simulink model "DA42HoloLensForwarder"  (R2021a)
settings: Solver=ode4  StartTime=0.0  StopTime=inf  FixedStep=0.001  RelTol=1e-3
undefined symbols (not defined in the file): Global_Sample_Time
libraries: simulink_extras x5, slrealtimeutilitieslib x2, dspnetwork x1
(part 3 of 5)

== system DA42HoloLensForwarder/FTD_Output_w_Multicast_XPCmod/Hardware_Switches/PanelAndLegroomSwitches/Decode_Flag1 ==
  Coded_Value : Inport
  Bitmask_Value : Constant  Value=hex2dec(Bitmask_Value)
  Bitwise Operator1 : S-Function  FunctionName=sfix_bitop  Parameters=UseBitMask,NumInputPorts,BitMask,BitMaskRealWorld,logicop  SFunctionDeploymentMode=off  EnableBusSupport=off  mask(Bitwise Operator){logicop=AND, UseBitMask=off, NumInputPorts=2, BitMask=bin2dec('11011001'), BitMaskRealWorld=Stored Integer}
      mask prompts: logicop "Operator:"; UseBitMask "Use bit mask ..."; NumInputPorts "Number of input ports:"; BitMask "Bit Mask"; BitMaskRealWorld "Treat mask as:"
      mask help: Perform the specified bitwise operation on the inputs. The output data type should represent zero exactly.
      mask init: same as DA42HoloLensForwarder/FTD_Output_w_Multicast_XPCmod/Hardware_Switches/MiscSwitches/Decode_Flag/Bitwise Operator1
      mask TypeOptions logicop: AND | OR | NAND | NOR | XOR | NOT
      mask Callback logicop: fixptdialog(gcbh)
      mask Callback UseBitMask: fixptdialog(gcbh)
      mask TypeOptions BitMaskRealWorld: Real World Value | Stored Integer
      mask Display: fprintf(['Bitwise\n',logicop,'\n',str])
  Data Type Conversion1 : DataTypeConversion  OutDataTypeStr=uint32
  Data Type Conversion2 : DataTypeConversion  OutDataTypeStr=double
  Data Type Conversion9 : DataTypeConversion  OutDataTypeStr=uint32
  Divide : Product  Inputs=*/
  Flag : Outport
  wires:
  Data Type Conversion2/1 -> Flag/1
  Divide/1 -> Data Type Conversion2/1
  Data Type Conversion1/1 -> Divide/2, Bitwise Operator1/2
  Data Type Conversion9/1 -> Bitwise Operator1/1
  Bitwise Operator1/1 -> Divide/1
  Bitmask_Value/1 -> Data Type Conversion1/1
  Coded_Value/1 -> Data Type Conversion9/1

== system DA42HoloLensForwarder/FTD_Output_w_Multicast_XPCmod/Hardware_Switches/PanelAndLegroomSwitches/Decode_Flag10 ==
  Coded_Value : Inport
  Bitmask_Value : Constant  Value=hex2dec(Bitmask_Value)
  Bitwise Operator1 : S-Function  FunctionName=sfix_bitop  Parameters=UseBitMask,NumInputPorts,BitMask,BitMaskRealWorld,logicop  SFunctionDeploymentMode=off  EnableBusSupport=off  mask(Bitwise Operator){logicop=AND, UseBitMask=off, NumInputPorts=2, BitMask=bin2dec('11011001'), BitMaskRealWorld=Stored Integer}
      mask prompts: logicop "Operator:"; UseBitMask "Use bit mask ..."; NumInputPorts "Number of input ports:"; BitMask "Bit Mask"; BitMaskRealWorld "Treat mask as:"
      mask help: Perform the specified bitwise operation on the inputs. The output data type should represent zero exactly.
      mask init: same as DA42HoloLensForwarder/FTD_Output_w_Multicast_XPCmod/Hardware_Switches/MiscSwitches/Decode_Flag/Bitwise Operator1
      mask TypeOptions logicop: AND | OR | NAND | NOR | XOR | NOT
      mask Callback logicop: fixptdialog(gcbh)
      mask Callback UseBitMask: fixptdialog(gcbh)
      mask TypeOptions BitMaskRealWorld: Real World Value | Stored Integer
      mask Display: fprintf(['Bitwise\n',logicop,'\n',str])
  Data Type Conversion1 : DataTypeConversion  OutDataTypeStr=uint32
  Data Type Conversion2 : DataTypeConversion  OutDataTypeStr=double
  Data Type Conversion9 : DataTypeConversion  OutDataTypeStr=uint32
  Divide : Product  Inputs=*/
  Flag : Outport
  wires:
  Data Type Conversion2/1 -> Flag/1
  Divide/1 -> Data Type Conversion2/1
  Data Type Conversion1/1 -> Divide/2, Bitwise Operator1/2
  Data Type Conversion9/1 -> Bitwise Operator1/1
  Bitwise Operator1/1 -> Divide/1
  Bitmask_Value/1 -> Data Type Conversion1/1
  Coded_Value/1 -> Data Type Conversion9/1

== system DA42HoloLensForwarder/FTD_Output_w_Multicast_XPCmod/Hardware_Switches/PanelAndLegroomSwitches/Decode_Flag11 ==
  Coded_Value : Inport
  Bitmask_Value : Constant  Value=hex2dec(Bitmask_Value)
  Bitwise Operator1 : S-Function  FunctionName=sfix_bitop  Parameters=UseBitMask,NumInputPorts,BitMask,BitMaskRealWorld,logicop  SFunctionDeploymentMode=off  EnableBusSupport=off  mask(Bitwise Operator){logicop=AND, UseBitMask=off, NumInputPorts=2, BitMask=bin2dec('11011001'), BitMaskRealWorld=Stored Integer}
      mask prompts: logicop "Operator:"; UseBitMask "Use bit mask ..."; NumInputPorts "Number of input ports:"; BitMask "Bit Mask"; BitMaskRealWorld "Treat mask as:"
      mask help: Perform the specified bitwise operation on the inputs. The output data type should represent zero exactly.
      mask init: same as DA42HoloLensForwarder/FTD_Output_w_Multicast_XPCmod/Hardware_Switches/MiscSwitches/Decode_Flag/Bitwise Operator1
      mask TypeOptions logicop: AND | OR | NAND | NOR | XOR | NOT
      mask Callback logicop: fixptdialog(gcbh)
      mask Callback UseBitMask: fixptdialog(gcbh)
      mask TypeOptions BitMaskRealWorld: Real World Value | Stored Integer
      mask Display: fprintf(['Bitwise\n',logicop,'\n',str])
  Data Type Conversion1 : DataTypeConversion  OutDataTypeStr=uint32
  Data Type Conversion2 : DataTypeConversion  OutDataTypeStr=double
  Data Type Conversion9 : DataTypeConversion  OutDataTypeStr=uint32
  Divide : Product  Inputs=*/
  Flag : Outport
  wires:
  Coded_Value/1 -> Data Type Conversion9/1
  Bitmask_Value/1 -> Data Type Conversion1/1
  Bitwise Operator1/1 -> Divide/1
  Data Type Conversion9/1 -> Bitwise Operator1/1
  Data Type Conversion1/1 -> Bitwise Operator1/2, Divide/2
  Divide/1 -> Data Type Conversion2/1
  Data Type Conversion2/1 -> Flag/1

== system DA42HoloLensForwarder/FTD_Output_w_Multicast_XPCmod/Hardware_Switches/PanelAndLegroomSwitches/Decode_Flag12 ==
  Coded_Value : Inport
  Bitmask_Value : Constant  Value=hex2dec(Bitmask_Value)
  Bitwise Operator1 : S-Function  FunctionName=sfix_bitop  Parameters=UseBitMask,NumInputPorts,BitMask,BitMaskRealWorld,logicop  SFunctionDeploymentMode=off  EnableBusSupport=off  mask(Bitwise Operator){logicop=AND, UseBitMask=off, NumInputPorts=2, BitMask=bin2dec('11011001'), BitMaskRealWorld=Stored Integer}
      mask prompts: logicop "Operator:"; UseBitMask "Use bit mask ..."; NumInputPorts "Number of input ports:"; BitMask "Bit Mask"; BitMaskRealWorld "Treat mask as:"
      mask help: Perform the specified bitwise operation on the inputs. The output data type should represent zero exactly.
      mask init: same as DA42HoloLensForwarder/FTD_Output_w_Multicast_XPCmod/Hardware_Switches/MiscSwitches/Decode_Flag/Bitwise Operator1
      mask TypeOptions logicop: AND | OR | NAND | NOR | XOR | NOT
      mask Callback logicop: fixptdialog(gcbh)
      mask Callback UseBitMask: fixptdialog(gcbh)
      mask TypeOptions BitMaskRealWorld: Real World Value | Stored Integer
      mask Display: fprintf(['Bitwise\n',logicop,'\n',str])
  Data Type Conversion1 : DataTypeConversion  OutDataTypeStr=uint32
  Data Type Conversion2 : DataTypeConversion  OutDataTypeStr=double
  Data Type Conversion9 : DataTypeConversion  OutDataTypeStr=uint32
  Divide : Product  Inputs=*/
  Flag : Outport
  wires:
  Data Type Conversion2/1 -> Flag/1
  Divide/1 -> Data Type Conversion2/1
  Data Type Conversion1/1 -> Divide/2, Bitwise Operator1/2
  Data Type Conversion9/1 -> Bitwise Operator1/1
  Bitwise Operator1/1 -> Divide/1
  Bitmask_Value/1 -> Data Type Conversion1/1
  Coded_Value/1 -> Data Type Conversion9/1

== system DA42HoloLensForwarder/FTD_Output_w_Multicast_XPCmod/Hardware_Switches/PanelAndLegroomSwitches/Decode_Flag13 ==
  Coded_Value : Inport
  Bitmask_Value : Constant  Value=hex2dec(Bitmask_Value)
  Bitwise Operator1 : S-Function  FunctionName=sfix_bitop  Parameters=UseBitMask,NumInputPorts,BitMask,BitMaskRealWorld,logicop  SFunctionDeploymentMode=off  EnableBusSupport=off  mask(Bitwise Operator){logicop=AND, UseBitMask=off, NumInputPorts=2, BitMask=bin2dec('11011001'), BitMaskRealWorld=Stored Integer}
      mask prompts: logicop "Operator:"; UseBitMask "Use bit mask ..."; NumInputPorts "Number of input ports:"; BitMask "Bit Mask"; BitMaskRealWorld "Treat mask as:"
      mask help: Perform the specified bitwise operation on the inputs. The output data type should represent zero exactly.
      mask init: same as DA42HoloLensForwarder/FTD_Output_w_Multicast_XPCmod/Hardware_Switches/MiscSwitches/Decode_Flag/Bitwise Operator1
      mask TypeOptions logicop: AND | OR | NAND | NOR | XOR | NOT
      mask Callback logicop: fixptdialog(gcbh)
      mask Callback UseBitMask: fixptdialog(gcbh)
      mask TypeOptions BitMaskRealWorld: Real World Value | Stored Integer
      mask Display: fprintf(['Bitwise\n',logicop,'\n',str])
  Data Type Conversion1 : DataTypeConversion  OutDataTypeStr=uint32
  Data Type Conversion2 : DataTypeConversion  OutDataTypeStr=double
  Data Type Conversion9 : DataTypeConversion  OutDataTypeStr=uint32
  Divide : Product  Inputs=*/
  Flag : Outport
  wires:
  Coded_Value/1 -> Data Type Conversion9/1
  Bitmask_Value/1 -> Data Type Conversion1/1
  Bitwise Operator1/1 -> Divide/1
  Data Type Conversion9/1 -> Bitwise Operator1/1
  Data Type Conversion1/1 -> Bitwise Operator1/2, Divide/2
  Divide/1 -> Data Type Conversion2/1
  Data Type Conversion2/1 -> Flag/1

== system DA42HoloLensForwarder/FTD_Output_w_Multicast_XPCmod/Hardware_Switches/PanelAndLegroomSwitches/Decode_Flag14 ==
  Coded_Value : Inport
  Bitmask_Value : Constant  Value=hex2dec(Bitmask_Value)
  Bitwise Operator1 : S-Function  FunctionName=sfix_bitop  Parameters=UseBitMask,NumInputPorts,BitMask,BitMaskRealWorld,logicop  SFunctionDeploymentMode=off  EnableBusSupport=off  mask(Bitwise Operator){logicop=AND, UseBitMask=off, NumInputPorts=2, BitMask=bin2dec('11011001'), BitMaskRealWorld=Stored Integer}
      mask prompts: logicop "Operator:"; UseBitMask "Use bit mask ..."; NumInputPorts "Number of input ports:"; BitMask "Bit Mask"; BitMaskRealWorld "Treat mask as:"
      mask help: Perform the specified bitwise operation on the inputs. The output data type should represent zero exactly.
      mask init: same as DA42HoloLensForwarder/FTD_Output_w_Multicast_XPCmod/Hardware_Switches/MiscSwitches/Decode_Flag/Bitwise Operator1
      mask TypeOptions logicop: AND | OR | NAND | NOR | XOR | NOT
      mask Callback logicop: fixptdialog(gcbh)
      mask Callback UseBitMask: fixptdialog(gcbh)
      mask TypeOptions BitMaskRealWorld: Real World Value | Stored Integer
      mask Display: fprintf(['Bitwise\n',logicop,'\n',str])
  Data Type Conversion1 : DataTypeConversion  OutDataTypeStr=uint32
  Data Type Conversion2 : DataTypeConversion  OutDataTypeStr=double
  Data Type Conversion9 : DataTypeConversion  OutDataTypeStr=uint32
  Divide : Product  Inputs=*/
  Flag : Outport
  wires:
  Coded_Value/1 -> Data Type Conversion9/1
  Bitmask_Value/1 -> Data Type Conversion1/1
  Bitwise Operator1/1 -> Divide/1
  Data Type Conversion9/1 -> Bitwise Operator1/1
  Data Type Conversion1/1 -> Bitwise Operator1/2, Divide/2
  Divide/1 -> Data Type Conversion2/1
  Data Type Conversion2/1 -> Flag/1

== system DA42HoloLensForwarder/FTD_Output_w_Multicast_XPCmod/Hardware_Switches/PanelAndLegroomSwitches/Decode_Flag15 ==
  Coded_Value : Inport
  Bitmask_Value : Constant  Value=hex2dec(Bitmask_Value)
  Bitwise Operator1 : S-Function  FunctionName=sfix_bitop  Parameters=UseBitMask,NumInputPorts,BitMask,BitMaskRealWorld,logicop  SFunctionDeploymentMode=off  EnableBusSupport=off  mask(Bitwise Operator){logicop=AND, UseBitMask=off, NumInputPorts=2, BitMask=bin2dec('11011001'), BitMaskRealWorld=Stored Integer}
      mask prompts: logicop "Operator:"; UseBitMask "Use bit mask ..."; NumInputPorts "Number of input ports:"; BitMask "Bit Mask"; BitMaskRealWorld "Treat mask as:"
      mask help: Perform the specified bitwise operation on the inputs. The output data type should represent zero exactly.
      mask init: same as DA42HoloLensForwarder/FTD_Output_w_Multicast_XPCmod/Hardware_Switches/MiscSwitches/Decode_Flag/Bitwise Operator1
      mask TypeOptions logicop: AND | OR | NAND | NOR | XOR | NOT
      mask Callback logicop: fixptdialog(gcbh)
      mask Callback UseBitMask: fixptdialog(gcbh)
      mask TypeOptions BitMaskRealWorld: Real World Value | Stored Integer
      mask Display: fprintf(['Bitwise\n',logicop,'\n',str])
  Data Type Conversion1 : DataTypeConversion  OutDataTypeStr=uint32
  Data Type Conversion2 : DataTypeConversion  OutDataTypeStr=double
  Data Type Conversion9 : DataTypeConversion  OutDataTypeStr=uint32
  Divide : Product  Inputs=*/
  Flag : Outport
  wires:
  Data Type Conversion2/1 -> Flag/1
  Divide/1 -> Data Type Conversion2/1
  Data Type Conversion1/1 -> Divide/2, Bitwise Operator1/2
  Data Type Conversion9/1 -> Bitwise Operator1/1
  Bitwise Operator1/1 -> Divide/1
  Bitmask_Value/1 -> Data Type Conversion1/1
  Coded_Value/1 -> Data Type Conversion9/1

== system DA42HoloLensForwarder/FTD_Output_w_Multicast_XPCmod/Hardware_Switches/PanelAndLegroomSwitches/Decode_Flag16 ==
  Coded_Value : Inport
  Bitmask_Value : Constant  Value=hex2dec(Bitmask_Value)
  Bitwise Operator1 : S-Function  FunctionName=sfix_bitop  Parameters=UseBitMask,NumInputPorts,BitMask,BitMaskRealWorld,logicop  SFunctionDeploymentMode=off  EnableBusSupport=off  mask(Bitwise Operator){logicop=AND, UseBitMask=off, NumInputPorts=2, BitMask=bin2dec('11011001'), BitMaskRealWorld=Stored Integer}
      mask prompts: logicop "Operator:"; UseBitMask "Use bit mask ..."; NumInputPorts "Number of input ports:"; BitMask "Bit Mask"; BitMaskRealWorld "Treat mask as:"
      mask help: Perform the specified bitwise operation on the inputs. The output data type should represent zero exactly.
      mask init: same as DA42HoloLensForwarder/FTD_Output_w_Multicast_XPCmod/Hardware_Switches/MiscSwitches/Decode_Flag/Bitwise Operator1
      mask TypeOptions logicop: AND | OR | NAND | NOR | XOR | NOT
      mask Callback logicop: fixptdialog(gcbh)
      mask Callback UseBitMask: fixptdialog(gcbh)
      mask TypeOptions BitMaskRealWorld: Real World Value | Stored Integer
      mask Display: fprintf(['Bitwise\n',logicop,'\n',str])
  Data Type Conversion1 : DataTypeConversion  OutDataTypeStr=uint32
  Data Type Conversion2 : DataTypeConversion  OutDataTypeStr=double
  Data Type Conversion9 : DataTypeConversion  OutDataTypeStr=uint32
  Divide : Product  Inputs=*/
  Flag : Outport
  wires:
  Coded_Value/1 -> Data Type Conversion9/1
  Bitmask_Value/1 -> Data Type Conversion1/1
  Bitwise Operator1/1 -> Divide/1
  Data Type Conversion9/1 -> Bitwise Operator1/1
  Data Type Conversion1/1 -> Bitwise Operator1/2, Divide/2
  Divide/1 -> Data Type Conversion2/1
  Data Type Conversion2/1 -> Flag/1

== system DA42HoloLensForwarder/FTD_Output_w_Multicast_XPCmod/Hardware_Switches/PanelAndLegroomSwitches/Decode_Flag17 ==
  Coded_Value : Inport
  Bitmask_Value : Constant  Value=hex2dec(Bitmask_Value)
  Bitwise Operator1 : S-Function  FunctionName=sfix_bitop  Parameters=UseBitMask,NumInputPorts,BitMask,BitMaskRealWorld,logicop  SFunctionDeploymentMode=off  EnableBusSupport=off  mask(Bitwise Operator){logicop=AND, UseBitMask=off, NumInputPorts=2, BitMask=bin2dec('11011001'), BitMaskRealWorld=Stored Integer}
      mask prompts: logicop "Operator:"; UseBitMask "Use bit mask ..."; NumInputPorts "Number of input ports:"; BitMask "Bit Mask"; BitMaskRealWorld "Treat mask as:"
      mask help: Perform the specified bitwise operation on the inputs. The output data type should represent zero exactly.
      mask init: same as DA42HoloLensForwarder/FTD_Output_w_Multicast_XPCmod/Hardware_Switches/MiscSwitches/Decode_Flag/Bitwise Operator1
      mask TypeOptions logicop: AND | OR | NAND | NOR | XOR | NOT
      mask Callback logicop: fixptdialog(gcbh)
      mask Callback UseBitMask: fixptdialog(gcbh)
      mask TypeOptions BitMaskRealWorld: Real World Value | Stored Integer
      mask Display: fprintf(['Bitwise\n',logicop,'\n',str])
  Data Type Conversion1 : DataTypeConversion  OutDataTypeStr=uint32
  Data Type Conversion2 : DataTypeConversion  OutDataTypeStr=double
  Data Type Conversion9 : DataTypeConversion  OutDataTypeStr=uint32
  Divide : Product  Inputs=*/
  Flag : Outport
  wires:
  Data Type Conversion2/1 -> Flag/1
  Divide/1 -> Data Type Conversion2/1
  Data Type Conversion1/1 -> Divide/2, Bitwise Operator1/2
  Data Type Conversion9/1 -> Bitwise Operator1/1
  Bitwise Operator1/1 -> Divide/1
  Bitmask_Value/1 -> Data Type Conversion1/1
  Coded_Value/1 -> Data Type Conversion9/1

== system DA42HoloLensForwarder/FTD_Output_w_Multicast_XPCmod/Hardware_Switches/PanelAndLegroomSwitches/Decode_Flag18 ==
  Coded_Value : Inport
  Bitmask_Value : Constant  Value=hex2dec(Bitmask_Value)
  Bitwise Operator1 : S-Function  FunctionName=sfix_bitop  Parameters=UseBitMask,NumInputPorts,BitMask,BitMaskRealWorld,logicop  SFunctionDeploymentMode=off  EnableBusSupport=off  mask(Bitwise Operator){logicop=AND, UseBitMask=off, NumInputPorts=2, BitMask=bin2dec('11011001'), BitMaskRealWorld=Stored Integer}
      mask prompts: logicop "Operator:"; UseBitMask "Use bit mask ..."; NumInputPorts "Number of input ports:"; BitMask "Bit Mask"; BitMaskRealWorld "Treat mask as:"
      mask help: Perform the specified bitwise operation on the inputs. The output data type should represent zero exactly.
      mask init: same as DA42HoloLensForwarder/FTD_Output_w_Multicast_XPCmod/Hardware_Switches/MiscSwitches/Decode_Flag/Bitwise Operator1
      mask TypeOptions logicop: AND | OR | NAND | NOR | XOR | NOT
      mask Callback logicop: fixptdialog(gcbh)
      mask Callback UseBitMask: fixptdialog(gcbh)
      mask TypeOptions BitMaskRealWorld: Real World Value | Stored Integer
      mask Display: fprintf(['Bitwise\n',logicop,'\n',str])
  Data Type Conversion1 : DataTypeConversion  OutDataTypeStr=uint32
  Data Type Conversion2 : DataTypeConversion  OutDataTypeStr=double
  Data Type Conversion9 : DataTypeConversion  OutDataTypeStr=uint32
  Divide : Product  Inputs=*/
  Flag : Outport
  wires:
  Data Type Conversion2/1 -> Flag/1
  Divide/1 -> Data Type Conversion2/1
  Data Type Conversion1/1 -> Divide/2, Bitwise Operator1/2
  Data Type Conversion9/1 -> Bitwise Operator1/1
  Bitwise Operator1/1 -> Divide/1
  Bitmask_Value/1 -> Data Type Conversion1/1
  Coded_Value/1 -> Data Type Conversion9/1

== system DA42HoloLensForwarder/FTD_Output_w_Multicast_XPCmod/Hardware_Switches/PanelAndLegroomSwitches/Decode_Flag19 ==
  Coded_Value : Inport
  Bitmask_Value : Constant  Value=hex2dec(Bitmask_Value)
  Bitwise Operator1 : S-Function  FunctionName=sfix_bitop  Parameters=UseBitMask,NumInputPorts,BitMask,BitMaskRealWorld,logicop  SFunctionDeploymentMode=off  EnableBusSupport=off  mask(Bitwise Operator){logicop=AND, UseBitMask=off, NumInputPorts=2, BitMask=bin2dec('11011001'), BitMaskRealWorld=Stored Integer}
      mask prompts: logicop "Operator:"; UseBitMask "Use bit mask ..."; NumInputPorts "Number of input ports:"; BitMask "Bit Mask"; BitMaskRealWorld "Treat mask as:"
      mask help: Perform the specified bitwise operation on the inputs. The output data type should represent zero exactly.
      mask init: same as DA42HoloLensForwarder/FTD_Output_w_Multicast_XPCmod/Hardware_Switches/MiscSwitches/Decode_Flag/Bitwise Operator1
      mask TypeOptions logicop: AND | OR | NAND | NOR | XOR | NOT
      mask Callback logicop: fixptdialog(gcbh)
      mask Callback UseBitMask: fixptdialog(gcbh)
      mask TypeOptions BitMaskRealWorld: Real World Value | Stored Integer
      mask Display: fprintf(['Bitwise\n',logicop,'\n',str])
  Data Type Conversion1 : DataTypeConversion  OutDataTypeStr=uint32
  Data Type Conversion2 : DataTypeConversion  OutDataTypeStr=double
  Data Type Conversion9 : DataTypeConversion  OutDataTypeStr=uint32
  Divide : Product  Inputs=*/
  Flag : Outport
  wires:
  Coded_Value/1 -> Data Type Conversion9/1
  Bitmask_Value/1 -> Data Type Conversion1/1
  Bitwise Operator1/1 -> Divide/1
  Data Type Conversion9/1 -> Bitwise Operator1/1
  Data Type Conversion1/1 -> Bitwise Operator1/2, Divide/2
  Divide/1 -> Data Type Conversion2/1
  Data Type Conversion2/1 -> Flag/1

== system DA42HoloLensForwarder/FTD_Output_w_Multicast_XPCmod/Hardware_Switches/PanelAndLegroomSwitches/Decode_Flag2 ==
  Coded_Value : Inport
  Bitmask_Value : Constant  Value=hex2dec(Bitmask_Value)
  Bitwise Operator1 : S-Function  FunctionName=sfix_bitop  Parameters=UseBitMask,NumInputPorts,BitMask,BitMaskRealWorld,logicop  SFunctionDeploymentMode=off  EnableBusSupport=off  mask(Bitwise Operator){logicop=AND, UseBitMask=off, NumInputPorts=2, BitMask=bin2dec('11011001'), BitMaskRealWorld=Stored Integer}
      mask prompts: logicop "Operator:"; UseBitMask "Use bit mask ..."; NumInputPorts "Number of input ports:"; BitMask "Bit Mask"; BitMaskRealWorld "Treat mask as:"
      mask help: Perform the specified bitwise operation on the inputs. The output data type should represent zero exactly.
      mask init: same as DA42HoloLensForwarder/FTD_Output_w_Multicast_XPCmod/Hardware_Switches/MiscSwitches/Decode_Flag/Bitwise Operator1
      mask TypeOptions logicop: AND | OR | NAND | NOR | XOR | NOT
      mask Callback logicop: fixptdialog(gcbh)
      mask Callback UseBitMask: fixptdialog(gcbh)
      mask TypeOptions BitMaskRealWorld: Real World Value | Stored Integer
      mask Display: fprintf(['Bitwise\n',logicop,'\n',str])
  Data Type Conversion1 : DataTypeConversion  OutDataTypeStr=uint32
  Data Type Conversion2 : DataTypeConversion  OutDataTypeStr=double
  Data Type Conversion9 : DataTypeConversion  OutDataTypeStr=uint32
  Divide : Product  Inputs=*/
  Flag : Outport
  wires:
  Data Type Conversion2/1 -> Flag/1
  Divide/1 -> Data Type Conversion2/1
  Data Type Conversion1/1 -> Divide/2, Bitwise Operator1/2
  Data Type Conversion9/1 -> Bitwise Operator1/1
  Bitwise Operator1/1 -> Divide/1
  Bitmask_Value/1 -> Data Type Conversion1/1
  Coded_Value/1 -> Data Type Conversion9/1

== system DA42HoloLensForwarder/FTD_Output_w_Multicast_XPCmod/Hardware_Switches/PanelAndLegroomSwitches/Decode_Flag20 ==
  Coded_Value : Inport
  Bitmask_Value : Constant  Value=hex2dec(Bitmask_Value)
  Bitwise Operator1 : S-Function  FunctionName=sfix_bitop  Parameters=UseBitMask,NumInputPorts,BitMask,BitMaskRealWorld,logicop  SFunctionDeploymentMode=off  EnableBusSupport=off  mask(Bitwise Operator){logicop=AND, UseBitMask=off, NumInputPorts=2, BitMask=bin2dec('11011001'), BitMaskRealWorld=Stored Integer}
      mask prompts: logicop "Operator:"; UseBitMask "Use bit mask ..."; NumInputPorts "Number of input ports:"; BitMask "Bit Mask"; BitMaskRealWorld "Treat mask as:"
      mask help: Perform the specified bitwise operation on the inputs. The output data type should represent zero exactly.
      mask init: same as DA42HoloLensForwarder/FTD_Output_w_Multicast_XPCmod/Hardware_Switches/MiscSwitches/Decode_Flag/Bitwise Operator1
      mask TypeOptions logicop: AND | OR | NAND | NOR | XOR | NOT
      mask Callback logicop: fixptdialog(gcbh)
      mask Callback UseBitMask: fixptdialog(gcbh)
      mask TypeOptions BitMaskRealWorld: Real World Value | Stored Integer
      mask Display: fprintf(['Bitwise\n',logicop,'\n',str])
  Data Type Conversion1 : DataTypeConversion  OutDataTypeStr=uint32
  Data Type Conversion2 : DataTypeConversion  OutDataTypeStr=double
  Data Type Conversion9 : DataTypeConversion  OutDataTypeStr=uint32
  Divide : Product  Inputs=*/
  Flag : Outport
  wires:
  Coded_Value/1 -> Data Type Conversion9/1
  Bitmask_Value/1 -> Data Type Conversion1/1
  Bitwise Operator1/1 -> Divide/1
  Data Type Conversion9/1 -> Bitwise Operator1/1
  Data Type Conversion1/1 -> Bitwise Operator1/2, Divide/2
  Divide/1 -> Data Type Conversion2/1
  Data Type Conversion2/1 -> Flag/1

== system DA42HoloLensForwarder/FTD_Output_w_Multicast_XPCmod/Hardware_Switches/PanelAndLegroomSwitches/Decode_Flag21 ==
  Coded_Value : Inport
  Bitmask_Value : Constant  Value=hex2dec(Bitmask_Value)
  Bitwise Operator1 : S-Function  FunctionName=sfix_bitop  Parameters=UseBitMask,NumInputPorts,BitMask,BitMaskRealWorld,logicop  SFunctionDeploymentMode=off  EnableBusSupport=off  mask(Bitwise Operator){logicop=AND, UseBitMask=off, NumInputPorts=2, BitMask=bin2dec('11011001'), BitMaskRealWorld=Stored Integer}
      mask prompts: logicop "Operator:"; UseBitMask "Use bit mask ..."; NumInputPorts "Number of input ports:"; BitMask "Bit Mask"; BitMaskRealWorld "Treat mask as:"
      mask help: Perform the specified bitwise operation on the inputs. The output data type should represent zero exactly.
      mask init: same as DA42HoloLensForwarder/FTD_Output_w_Multicast_XPCmod/Hardware_Switches/MiscSwitches/Decode_Flag/Bitwise Operator1
      mask TypeOptions logicop: AND | OR | NAND | NOR | XOR | NOT
      mask Callback logicop: fixptdialog(gcbh)
      mask Callback UseBitMask: fixptdialog(gcbh)
      mask TypeOptions BitMaskRealWorld: Real World Value | Stored Integer
      mask Display: fprintf(['Bitwise\n',logicop,'\n',str])
  Data Type Conversion1 : DataTypeConversion  OutDataTypeStr=uint32
  Data Type Conversion2 : DataTypeConversion  OutDataTypeStr=double
  Data Type Conversion9 : DataTypeConversion  OutDataTypeStr=uint32
  Divide : Product  Inputs=*/
  Flag : Outport
  wires:
  Data Type Conversion2/1 -> Flag/1
  Divide/1 -> Data Type Conversion2/1
  Data Type Conversion1/1 -> Divide/2, Bitwise Operator1/2
  Data Type Conversion9/1 -> Bitwise Operator1/1
  Bitwise Operator1/1 -> Divide/1
  Bitmask_Value/1 -> Data Type Conversion1/1
  Coded_Value/1 -> Data Type Conversion9/1

== system DA42HoloLensForwarder/FTD_Output_w_Multicast_XPCmod/Hardware_Switches/PanelAndLegroomSwitches/Decode_Flag22 ==
  Coded_Value : Inport
  Bitmask_Value : Constant  Value=hex2dec(Bitmask_Value)
  Bitwise Operator1 : S-Function  FunctionName=sfix_bitop  Parameters=UseBitMask,NumInputPorts,BitMask,BitMaskRealWorld,logicop  SFunctionDeploymentMode=off  EnableBusSupport=off  mask(Bitwise Operator){logicop=AND, UseBitMask=off, NumInputPorts=2, BitMask=bin2dec('11011001'), BitMaskRealWorld=Stored Integer}
      mask prompts: logicop "Operator:"; UseBitMask "Use bit mask ..."; NumInputPorts "Number of input ports:"; BitMask "Bit Mask"; BitMaskRealWorld "Treat mask as:"
      mask help: Perform the specified bitwise operation on the inputs. The output data type should represent zero exactly.
      mask init: same as DA42HoloLensForwarder/FTD_Output_w_Multicast_XPCmod/Hardware_Switches/MiscSwitches/Decode_Flag/Bitwise Operator1
      mask TypeOptions logicop: AND | OR | NAND | NOR | XOR | NOT
      mask Callback logicop: fixptdialog(gcbh)
      mask Callback UseBitMask: fixptdialog(gcbh)
      mask TypeOptions BitMaskRealWorld: Real World Value | Stored Integer
      mask Display: fprintf(['Bitwise\n',logicop,'\n',str])
  Data Type Conversion1 : DataTypeConversion  OutDataTypeStr=uint32
  Data Type Conversion2 : DataTypeConversion  OutDataTypeStr=double
  Data Type Conversion9 : DataTypeConversion  OutDataTypeStr=uint32
  Divide : Product  Inputs=*/
  Flag : Outport
  wires:
  Data Type Conversion2/1 -> Flag/1
  Divide/1 -> Data Type Conversion2/1
  Data Type Conversion1/1 -> Divide/2, Bitwise Operator1/2
  Data Type Conversion9/1 -> Bitwise Operator1/1
  Bitwise Operator1/1 -> Divide/1
  Bitmask_Value/1 -> Data Type Conversion1/1
  Coded_Value/1 -> Data Type Conversion9/1

== system DA42HoloLensForwarder/FTD_Output_w_Multicast_XPCmod/Hardware_Switches/PanelAndLegroomSwitches/Decode_Flag23 ==
  Coded_Value : Inport
  Bitmask_Value : Constant  Value=hex2dec(Bitmask_Value)
  Bitwise Operator1 : S-Function  FunctionName=sfix_bitop  Parameters=UseBitMask,NumInputPorts,BitMask,BitMaskRealWorld,logicop  SFunctionDeploymentMode=off  EnableBusSupport=off  mask(Bitwise Operator){logicop=AND, UseBitMask=off, NumInputPorts=2, BitMask=bin2dec('11011001'), BitMaskRealWorld=Stored Integer}
      mask prompts: logicop "Operator:"; UseBitMask "Use bit mask ..."; NumInputPorts "Number of input ports:"; BitMask "Bit Mask"; BitMaskRealWorld "Treat mask as:"
      mask help: Perform the specified bitwise operation on the inputs. The output data type should represent zero exactly.
      mask init: same as DA42HoloLensForwarder/FTD_Output_w_Multicast_XPCmod/Hardware_Switches/MiscSwitches/Decode_Flag/Bitwise Operator1
      mask TypeOptions logicop: AND | OR | NAND | NOR | XOR | NOT
      mask Callback logicop: fixptdialog(gcbh)
      mask Callback UseBitMask: fixptdialog(gcbh)
      mask TypeOptions BitMaskRealWorld: Real World Value | Stored Integer
      mask Display: fprintf(['Bitwise\n',logicop,'\n',str])
  Data Type Conversion1 : DataTypeConversion  OutDataTypeStr=uint32
  Data Type Conversion2 : DataTypeConversion  OutDataTypeStr=double
  Data Type Conversion9 : DataTypeConversion  OutDataTypeStr=uint32
  Divide : Product  Inputs=*/
  Flag : Outport
  wires:
  Coded_Value/1 -> Data Type Conversion9/1
  Bitmask_Value/1 -> Data Type Conversion1/1
  Bitwise Operator1/1 -> Divide/1
  Data Type Conversion9/1 -> Bitwise Operator1/1
  Data Type Conversion1/1 -> Bitwise Operator1/2, Divide/2
  Divide/1 -> Data Type Conversion2/1
  Data Type Conversion2/1 -> Flag/1

== system DA42HoloLensForwarder/FTD_Output_w_Multicast_XPCmod/Hardware_Switches/PanelAndLegroomSwitches/Decode_Flag24 ==
  Coded_Value : Inport
  Bitmask_Value : Constant  Value=hex2dec(Bitmask_Value)
  Bitwise Operator1 : S-Function  FunctionName=sfix_bitop  Parameters=UseBitMask,NumInputPorts,BitMask,BitMaskRealWorld,logicop  SFunctionDeploymentMode=off  EnableBusSupport=off  mask(Bitwise Operator){logicop=AND, UseBitMask=off, NumInputPorts=2, BitMask=bin2dec('11011001'), BitMaskRealWorld=Stored Integer}
      mask prompts: logicop "Operator:"; UseBitMask "Use bit mask ..."; NumInputPorts "Number of input ports:"; BitMask "Bit Mask"; BitMaskRealWorld "Treat mask as:"
      mask help: Perform the specified bitwise operation on the inputs. The output data type should represent zero exactly.
      mask init: same as DA42HoloLensForwarder/FTD_Output_w_Multicast_XPCmod/Hardware_Switches/MiscSwitches/Decode_Flag/Bitwise Operator1
      mask TypeOptions logicop: AND | OR | NAND | NOR | XOR | NOT
      mask Callback logicop: fixptdialog(gcbh)
      mask Callback UseBitMask: fixptdialog(gcbh)
      mask TypeOptions BitMaskRealWorld: Real World Value | Stored Integer
      mask Display: fprintf(['Bitwise\n',logicop,'\n',str])
  Data Type Conversion1 : DataTypeConversion  OutDataTypeStr=uint32
  Data Type Conversion2 : DataTypeConversion  OutDataTypeStr=double
  Data Type Conversion9 : DataTypeConversion  OutDataTypeStr=uint32
  Divide : Product  Inputs=*/
  Flag : Outport
  wires:
  Data Type Conversion2/1 -> Flag/1
  Divide/1 -> Data Type Conversion2/1
  Data Type Conversion1/1 -> Divide/2, Bitwise Operator1/2
  Data Type Conversion9/1 -> Bitwise Operator1/1
  Bitwise Operator1/1 -> Divide/1
  Bitmask_Value/1 -> Data Type Conversion1/1
  Coded_Value/1 -> Data Type Conversion9/1
